simulink model "staubli_simulink"  (R2020b)
settings: Solver=VariableStepAuto  StartTime=0.0  StopTime=10.0  RelTol=1e-3
libraries: dsppolyfun x2, simulink x2
settings Model: Creator=이해구  LastModifiedBy=이해구

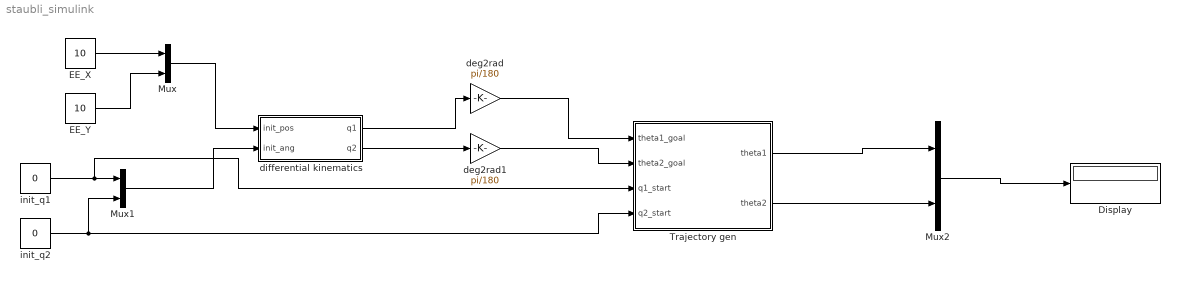
== system staubli_simulink ==
  Display : Display
  EE_X : Constant  Value=10
  EE_Y : Constant  Value=10
  Mux : Mux  Inputs=2
  Mux1 : Mux  Inputs=2
  Mux2 : Mux  Inputs=2
  Trajectory gen : Subsystem
  deg2rad : Gain  Gain=pi/180
  deg2rad1 : Gain  Gain=pi/180
  differential kinematics : Subsystem
  init_q1 : Constant  Value=0
  init_q2 : Constant  Value=0
  wires:
  Mux1/1 -> differential kinematics/2(init_ang)
  Trajectory gen/1(theta1) -> Mux2/1
  Mux/1 -> differential kinematics/1(init_pos)
  EE_X/1 -> Mux/1
  EE_Y/1 -> Mux/2
  Trajectory gen/2(theta2) -> Mux2/2
  Mux2/1 -> Display/1
  deg2rad/1 -> Trajectory gen/1("theta1_goal ")
  deg2rad1/1 -> Trajectory gen/2(theta2_goal)
  init_q1/1 -> Trajectory gen/3(q1_start), Mux1/1
  init_q2/1 -> Trajectory gen/4(q2_start), Mux1/2
  differential kinematics/1(q1) -> deg2rad/1
  differential kinematics/2(q2) -> deg2rad1/1

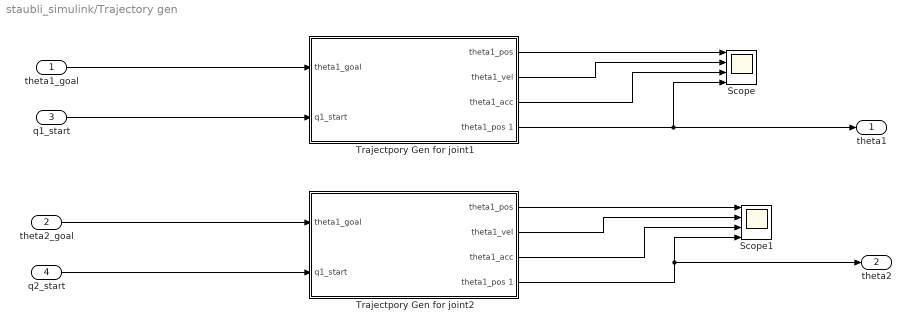
== system staubli_simulink/Trajectory gen ==
  "theta1_goal " : Inport
  theta2_goal : Inport  Port=2
  q1_start : Inport  Port=3
  q2_start : Inport  Port=4
  Scope : Scope  NumInputPorts=4
  Scope1 : Scope  NumInputPorts=4
  Trajectpory Gen for joint1 : Subsystem
  Trajectpory Gen for joint2 : Subsystem
  theta1 : Outport
  theta2 : Outport  Port=2
  wires:
  "theta1_goal "/1 -> Trajectpory Gen for joint1/1("theta1_goal ")
  q1_start/1 -> Trajectpory Gen for joint1/2("q1_start ")
  Trajectpory Gen for joint1/1("theta1_pos ") -> Scope/1
  Trajectpory Gen for joint1/2("theta1_vel ") -> Scope/2
  Trajectpory Gen for joint1/3("theta1_acc ") -> Scope/3
  Trajectpory Gen for joint1/4(theta1_pos 1) -> Scope/4, theta1/1
  Trajectpory Gen for joint2/1("theta1_pos ") -> Scope1/1
  Trajectpory Gen for joint2/2("theta1_vel ") -> Scope1/2
  Trajectpory Gen for joint2/3("theta1_acc ") -> Scope1/3
  Trajectpory Gen for joint2/4(theta1_pos 1) -> theta2/1, Scope1/4
  theta2_goal/1 -> Trajectpory Gen for joint2/1("theta1_goal ")
  q2_start/1 -> Trajectpory Gen for joint2/2("q1_start ")

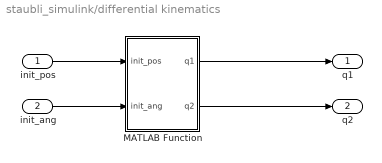
== system staubli_simulink/differential kinematics ==
  init_pos : Inport
  init_ang : Inport  Port=2
  MATLAB Function : MATLAB Function  TreatAsAtomicUnit=on
  q1 : Outport
  q2 : Outport  Port=2
  wires:
  init_pos/1 -> MATLAB Function/1(init_pos)
  MATLAB Function/1(q1) -> q1/1
  init_ang/1 -> MATLAB Function/2(init_ang)
  MATLAB Function/2(q2) -> q2/1

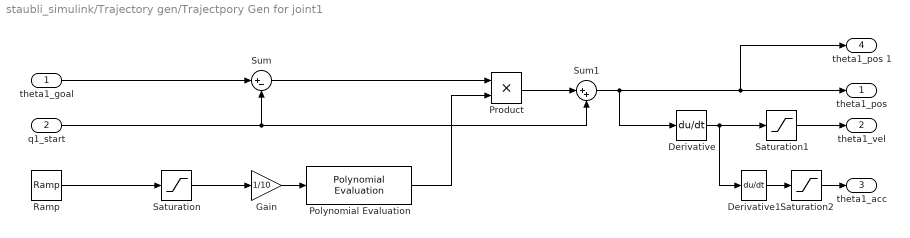
== system staubli_simulink/Trajectory gen/Trajectpory Gen for joint1 ==
  "theta1_goal " : Inport
  "q1_start " : Inport  Port=2
  Derivative : Derivative
  Derivative1 : Derivative
  Gain : Gain  Gain=1/10
  Polynomial Evaluation : dsppolyfun/Polynomial Evaluation  useConstCoeffs=on  constCoeffs=[6 -15 10 0 0 0]
      settings: SourceProductBaseCode=DS
  Product : Product
  Ramp : simulink/Sources/Ramp  slope=1  start=0  InitialOutput=0
  Saturation : Saturate  UpperLimit=10  LowerLimit=-10
  Saturation1 : Saturate
  Saturation2 : Saturate
  Sum : Sum  Inputs=|+-
  Sum1 : Sum  Inputs=|++
  "theta1_pos " : Outport  VectorParamsAs1DForOutWhenUnconnected=off
  "theta1_vel " : Outport  Port=2  VectorParamsAs1DForOutWhenUnconnected=off
  "theta1_acc " : Outport  Port=3  VectorParamsAs1DForOutWhenUnconnected=off
  theta1_pos 1 : Outport  Port=4  VectorParamsAs1DForOutWhenUnconnected=off
  wires:
  "q1_start "/1 -> Sum1/2, Sum/2
  Sum/1 -> Product/1
  "theta1_goal "/1 -> Sum/1
  Sum1/1 -> Derivative/1, theta1_pos 1/1, "theta1_pos "/1
  Derivative1/1 -> Saturation2/1
  Saturation1/1 -> "theta1_vel "/1
  Gain/1 -> Polynomial Evaluation/1
  Product/1 -> Sum1/1
  Polynomial Evaluation/1 -> Product/2
  Saturation2/1 -> "theta1_acc "/1
  Saturation/1 -> Gain/1
  Ramp/1 -> Saturation/1
  Derivative/1 -> Derivative1/1, Saturation1/1

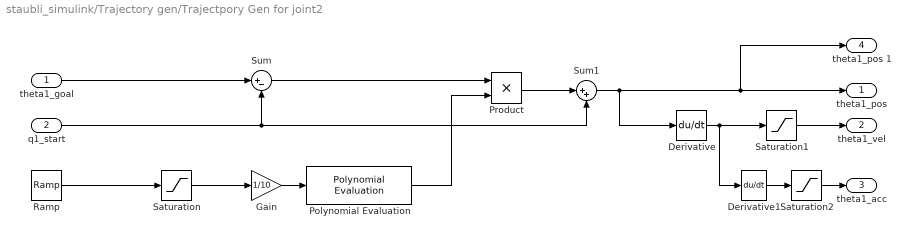
== system staubli_simulink/Trajectory gen/Trajectpory Gen for joint2 ==
  "theta1_goal " : Inport
  "q1_start " : Inport  Port=2
  Derivative : Derivative
  Derivative1 : Derivative
  Gain : Gain  Gain=1/10
  Polynomial Evaluation : dsppolyfun/Polynomial Evaluation  useConstCoeffs=on  constCoeffs=[6 -15 10 0 0 0]
      settings: SourceProductBaseCode=DS
  Product : Product
  Ramp : simulink/Sources/Ramp  slope=1  start=0  InitialOutput=0
  Saturation : Saturate  UpperLimit=10  LowerLimit=-10
  Saturation1 : Saturate
  Saturation2 : Saturate
  Sum : Sum  Inputs=|+-
  Sum1 : Sum  Inputs=|++
  "theta1_pos " : Outport  VectorParamsAs1DForOutWhenUnconnected=off
  "theta1_vel " : Outport  Port=2  VectorParamsAs1DForOutWhenUnconnected=off
  "theta1_acc " : Outport  Port=3  VectorParamsAs1DForOutWhenUnconnected=off
  theta1_pos 1 : Outport  Port=4  VectorParamsAs1DForOutWhenUnconnected=off
  wires:
  "q1_start "/1 -> Sum1/2, Sum/2
  Sum/1 -> Product/1
  "theta1_goal "/1 -> Sum/1
  Sum1/1 -> Derivative/1, theta1_pos 1/1, "theta1_pos "/1
  Derivative1/1 -> Saturation2/1
  Saturation1/1 -> "theta1_vel "/1
  Gain/1 -> Polynomial Evaluation/1
  Product/1 -> Sum1/1
  Polynomial Evaluation/1 -> Product/2
  Saturation2/1 -> "theta1_acc "/1
  Saturation/1 -> Gain/1
  Ramp/1 -> Saturation/1
  Derivative/1 -> Derivative1/1, Saturation1/1

== matlab function staubli_simulink/differential kinematics/MATLAB Function ==
  data: init_pos input; q1 output; init_ang input; q2 output
function [q1,q2]= jacobian(init_pos, init_ang)
theta1=init_ang(1);d1=0;a1=10;alpha1=0; %parameter link1
theta2=init_ang(2);d2=0;a2=10;alpha2=0; %parameter link2
%theta3=0;d3=0;a3=5;alpha3=0; %parameter link3

deltatheta1=0;deltatheta2=0; %theta1,2,3 velocity
Xc=init_pos(1);Yc=init_pos(2);
b=0;
orin_error = 0;
count =0;
while b==0
    count= count+1;
    if(count > 100)
        b=1;
        count =0;
    end
    theta1=theta1+deltatheta1/2;
    theta2=theta2+deltatheta2/2;
    %theta3=theta3+deltatheta3/2; %360-theta1-theta2;
    T01=[cosd(theta1) -sind(theta1)*cosd(alpha1) sind(theta1)*sind(alpha1) a1*cosd(theta1);
         sind(theta1) cosd(theta1)*cosd(alpha1)  -cosd(theta1)*sind(alpha1) a1*sind(theta1);
         0,sind(alpha1),cosd(alpha1),d1;
         0,0,0,1];
    T12=[cosd(theta2) -sind(theta2)*cosd(alpha2) sind(theta2)*sind(alpha2) a2*cosd(theta2);
         sind(theta2) cosd(theta2)*cosd(alpha2)  -cosd(theta2)*sind(alpha2) a2*sind(theta2);
         0,sind(alpha2),cosd(alpha2),d2;
         0,0,0,1];
%         disp('T01: '); disp(T01)
%         disp('T02: '); disp(T12)
    %T23=DHmatrix(theta3,d3,a3,alpha3);
    T02=T01*T12;
    P0=[0 0];
    P1=transpose(T01(1:2,4));
    P2=transpose(T02(1:2,4));
    %Linear velocity jacobian
    %Prismatic: Jv = zi-1
    %Revolute: Jv = zi-1 x (on - oi-1)
    Z0=[0;0;1];O=[0;0;0];O2=T02(1:3,4);
    Jv1=cross(Z0,(O2-O));
    Z1=T01(1:3,3);O1=T01(1:3,4);
    Jv2=cross(Z1,(O2-O1));
    %Z3=T12(1:3,3);O2=T12(1:3,4);
    %Jv3=cross(Z1,(O3-O2));
    Jv=[Jv1 Jv2];
    %disp('Jv:'); disp(Jv);

    Xinit=P2(1,1);Yinit=P2(1,2);
    Xend=Xc;Yend=Yc; 
    Xspeed=(Xend-Xinit);
    Yspeed=(Yend-Yinit);
    %Pseudoinverse Jacobian
    thetadot=pinv(Jv)*[Xspeed;Yspeed;0];
    OrinEnd=atan2d(Yend,Xend);
    Orininit=atan2d(Yinit,Xinit);
    dis_error=sqrt(Xend^2+Yend^2)- sqrt(Xinit^2+Yinit^2)
    orin_error=OrinEnd-Orininit
    if abs(dis_error)<=0.02 & abs(orin_error)<=2
        b=1;
    end
    theta1dot=thetadot(1,1);
    theta2dot=thetadot(2,1);

    deltatheta1=rad2deg(theta1dot);
    deltatheta2=rad2deg(theta2dot);
    deltatheta=[deltatheta1;deltatheta2];
end
q1 = theta1;
q2 = theta2;
